simulink model "task1"  (R2024a)
settings: Solver=VariableStepAuto  StartTime=0.0  StopTime=10.0  RelTol=1e-3
settings Model: Creator=sizgr  LastModifiedBy=sizgr

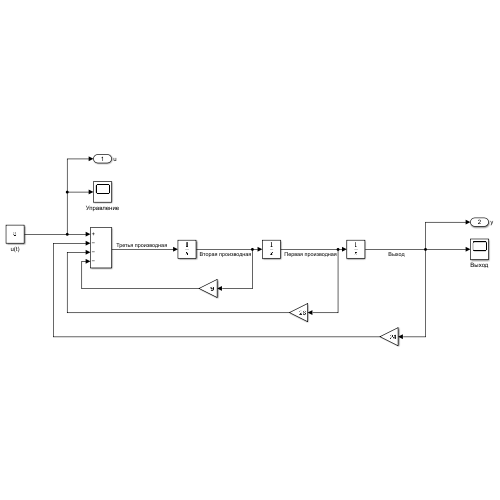
[thumbnail: Simulink's stored preview of the top-level diagram]
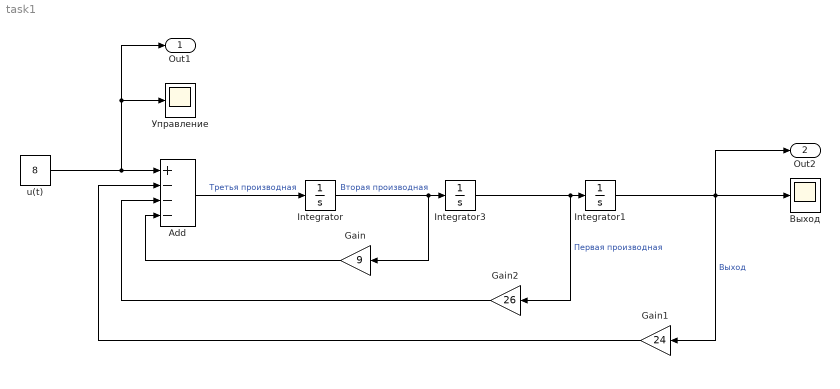
== system task1 ==
  Add : Sum  Inputs=+---
  Gain : Gain  Gain=9
  Gain1 : Gain  Gain=24
  Gain2 : Gain  Gain=26
  Integrator : Integrator
  Integrator1 : Integrator
  Integrator3 : Integrator
  u(t) : Constant  Value=8
  Выход : Scope
  Управление : Scope
  Out1 : Outport  SignalName=u
  Out2 : Outport  Port=2  SignalName=y
  wires:
  u(t)/1 -> Out1/1, Управление/1, Add/1
  Add/1 -> Integrator/1  "Третья производная"
  Integrator/1 -> Gain/1, Integrator3/1  "Вторая производная"
  Integrator3/1 -> Gain2/1, Integrator1/1  "Первая производная"
  Gain/1 -> Add/4
  Gain2/1 -> Add/3
  Integrator1/1 -> Out2/1, Выход/1, Gain1/1  "Выход"
  Gain1/1 -> Add/2
